simulink model "Sir_"  (R2015a)
settings: Solver=ode15s  StartTime=0.0  StopTime=10.0  RelTol=1e-3
libraries: fl_lib x20, elec_lib x9, nesl_utility x4, slctrlblks x1
settings Model: Creator=Ferdous  LastModifiedBy=joypc

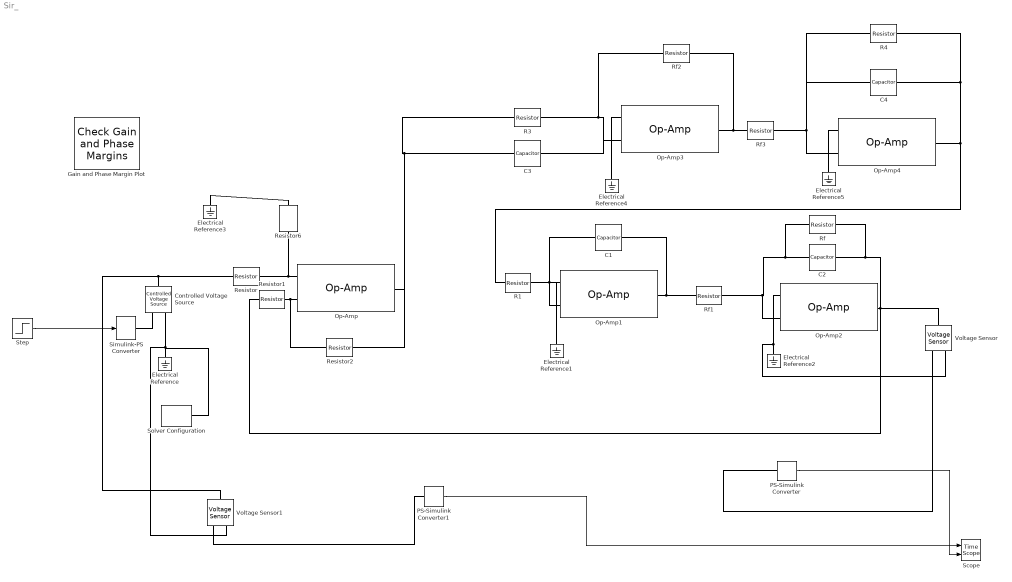
== system Sir_ ==
  C1 : fl_lib/Electrical/Electrical Elements/Capacitor  c=1e-6 F  r=1e-6 Ohm  g=0 1/Ohm  i_specify=off  i_priority=High  i=0 A  v_specify=off  v_priority=High  v=0 V  vc_specify=off  vc_priority=High  vc=0 V
  C2 : fl_lib/Electrical/Electrical Elements/Capacitor  c=0.122255367 F  r=1e-6 Ohm  g=0 1/Ohm  i_specify=off  i_priority=High  i=0 A  v_specify=off  v_priority=High  v=0 V  vc_specify=off  vc_priority=High  vc=0 V
  C3 : fl_lib/Electrical/Electrical Elements/Capacitor  c=2.51154 F  r=1e-6 Ohm  g=0 1/Ohm  i_specify=off  i_priority=High  i=0 A  v_specify=off  v_priority=High  v=0 V  vc_specify=off  vc_priority=High  vc=0 V
  C4 : fl_lib/Electrical/Electrical Elements/Capacitor  c=1.56 F  r=1e-6 Ohm  g=0 1/Ohm  i_specify=off  i_priority=High  i=0 A  v_specify=off  v_priority=High  v=0 V  vc_specify=off  vc_priority=High  vc=0 V
  Controlled Voltage Source : fl_lib/Electrical/Electrical Sources/Controlled Voltage Source
  Electrical Reference{,1..5} (6 alike) : fl_lib/Electrical/Electrical Elements/Electrical Reference
  Gain and Phase Margin Plot : slctrlblks/Model Verification/Check Gain and Phase Margins  InstantiateOnLoad=on  SaveOperatingPoints=off  LinearizationIOs={'/Step', 1, 'in', 'off', '';'/PS-Simulink Converter', 1, 'out', 'on', ''}  LinearizeAt=SnapshotTimes  SnapshotTimes=[0]  TriggerType=rising  SampleTime=auto  RateConversionMethod=zoh  PreWarpFreq=10  UseExactDelayModel=off  UseFullBlockNameLabels=off  UseBusSignalLabels=off  enabled=on  stopWhenAssertionFail=off  export=off  ViewDlgPos=[100 200 510 390]  LaunchViewOnOpen=off  OpenViewOnLoad=off  FrequencyUnits=rad/s  MagnitudeUnits=dB  PhaseUnits=deg  TimeUnits=seconds  EnableMargins=off  GainMargin=[]  PhaseMargin=[]  PlotType=bode  FeedbackSign=-1
      settings: SaveToWorkspace=off  SaveName=sys
  Op-Amp{,1..4} (5 alike) : fl_lib/Electrical/Electrical Elements/Op-Amp  outI_specify=off  outI_priority=High  outI=0 A
  PS-Simulink Converter : nesl_utility/PS-Simulink Converter  PhysicalDomain=network_engine_domain  SubClassName=ps_output  LeftPortType=input  RightPortType=output  PseudoPeriodic=off  Frequencies=[]  Unit=1  AffineConversion=off
  PS-Simulink Converter1 : nesl_utility/PS-Simulink Converter  PhysicalDomain=network_engine_domain  SubClassName=ps_output  LeftPortType=input  RightPortType=output  PseudoPeriodic=off  Frequencies=[]  Unit=1  AffineConversion=off
  R1 : elec_lib/Passive Devices/Resistor  R=1 kOhm  noise_mode=0  Tdevice=25 C  sample_time=0.001 s  repeatability=1  auto_seed=2279758131  user_seed=0
  R3 : elec_lib/Passive Devices/Resistor  R=0.995584 Ohm  noise_mode=0  Tdevice=25 C  sample_time=0.001 s  repeatability=1  auto_seed=1450493821  user_seed=0
  "R4 " : elec_lib/Passive Devices/Resistor  R=2.58816 Ohm  noise_mode=0  Tdevice=25 C  sample_time=0.001 s  repeatability=1  auto_seed=3865701835  user_seed=0
  Resistor : fl_lib/Electrical/Electrical Elements/Resistor  R=1 kOhm  i_specify=off  i_priority=High  i=0 A  v_specify=off  v_priority=High  v=0 V
  Resistor1 : fl_lib/Electrical/Electrical Elements/Resistor  R=1 kOhm  i_specify=off  i_priority=High  i=0 A  v_specify=off  v_priority=High  v=0 V
  Resistor2 : elec_lib/Passive Devices/Resistor  R=1 kOhm  noise_mode=0  Tdevice=25 C  sample_time=0.001 s  repeatability=1  auto_seed=1092133643  user_seed=0
  Resistor6 : elec_lib/Passive Devices/Resistor  R=1 kOhm  noise_mode=0  Tdevice=25 C  sample_time=0.001 s  repeatability=1  auto_seed=1585902849  user_seed=0
  Rf : elec_lib/Passive Devices/Resistor  R=5.107142857 Ohm  noise_mode=0  Tdevice=25 C  sample_time=0.001 s  repeatability=1  auto_seed=654458608  user_seed=0
  Rf1 : elec_lib/Passive Devices/Resistor  R=1 kOhm  noise_mode=0  Tdevice=25 C  sample_time=0.001 s  repeatability=1  auto_seed=3346497771  user_seed=0
  Rf2 : elec_lib/Passive Devices/Resistor  R=1 Ohm  noise_mode=0  Tdevice=25 C  sample_time=0.001 s  repeatability=1  auto_seed=1585902849  user_seed=0
  Rf3 : elec_lib/Passive Devices/Resistor  R=1 Ohm  noise_mode=0  Tdevice=25 C  sample_time=0.001 s  repeatability=1  auto_seed=477612198  user_seed=0
  Scope : TimeScope  NumInputPorts=2
  Simulink-PS Converter : nesl_utility/Simulink-PS Converter  PhysicalDomain=network_engine_domain  SubClassName=ps_input  LeftPortType=input  RightPortType=output  PseudoPeriodic=off  Frequencies=[]  NoiseDistribution=none  NoiseParameters=[]  Unit=1  AffineConversion=off  InputFiltering=off  SimscapeFilterOrder=1  InputFilterTimeConstant=0.001  UdotUserProvided=1
  Solver Configuration : nesl_utility/Solver Configuration  PhysicalDomain=network_engine_domain  SubClassName=solver  LeftPortType=input  RightPortType=generic  Accelerate=off  Tones=[]  Harmonics=[]  SimulateNoise=off  Profile=off  UseLocalSampling=off  EnableSwitchedLinearOptims=on  FrequencyDomain=off  UseCCode=off  RelTol=0.001  AbsTol=1e-06  MinStep=1e-09  ToWorkspace=off  RevertToSquareIcSolve=off  NumHomotopyIterations=100  DoDC=off  ResidualTolerance=1e-09  UseLocalSolver=off  LocalSolverChoice=NE_BACKWARD_EULER_ADVANCER  LocalSolverSampleTime=0.001  DoFixedCost=off  MaxNonlinIter=3  MaxModeIter=2  LinearAlgebra=Sparse  DelaysMemoryBudget=1024  AutomaticFiltering=on  FilteringTimeConstant=0.001
  Step : Step  SampleTime=0
  Voltage Sensor : fl_lib/Electrical/Electrical Sensors/Voltage Sensor
  Voltage Sensor1 : fl_lib/Electrical/Electrical Sensors/Voltage Sensor
  wires:
  Step/1 -> Simulink-PS Converter/1
  PS-Simulink Converter1/1 -> Scope/1
  PS-Simulink Converter/1 -> Scope/2
  connections:
  Resistor/RConn1 -- Resistor6/LConn1 -- Op-Amp/LConn1
  Resistor1/LConn1 -- Resistor2/LConn1 -- Op-Amp/LConn2
  Controlled Voltage Source/LConn1 -- Voltage Sensor1/LConn1 -- Resistor/LConn1
  Electrical Reference/LConn1 -- Controlled Voltage Source/RConn2 -- Solver Configuration/RConn1 -- Voltage Sensor1/RConn2
  Simulink-PS Converter/RConn1 -- Controlled Voltage Source/RConn1
  R1/RConn1 -- C1/LConn1 -- Op-Amp1/LConn2
  Rf1/LConn1 -- Op-Amp1/RConn1 -- C1/RConn1
  Rf1/RConn1 -- Op-Amp2/LConn2 -- Rf/LConn1 -- C2/LConn1
  C2/RConn1 -- Rf/RConn1 -- Voltage Sensor/LConn1 -- Op-Amp2/RConn1 -- Resistor1/RConn1
  Op-Amp1/LConn1 -- Electrical Reference1/LConn1
  Electrical Reference2/LConn1 -- Voltage Sensor/RConn2 -- Op-Amp2/LConn1
  Voltage Sensor1/RConn1 -- PS-Simulink Converter1/LConn1
  Voltage Sensor/RConn1 -- PS-Simulink Converter/LConn1
  Electrical Reference3/LConn1 -- Resistor6/RConn1
  Rf2/LConn1 -- R3/RConn1 -- Op-Amp3/LConn2 -- C3/RConn1
  Op-Amp3/RConn1 -- Rf2/RConn1 -- Rf3/LConn1
  Rf3/RConn1 -- Op-Amp4/LConn2 -- "R4 "/LConn1 -- C4/LConn1
  "R4 "/RConn1 -- C4/RConn1 -- R1/LConn1 -- Op-Amp4/RConn1
  C3/LConn1 -- Resistor2/RConn1 -- Op-Amp/RConn1 -- R3/LConn1
  Op-Amp4/LConn1 -- Electrical Reference5/LConn1
  Op-Amp3/LConn1 -- Electrical Reference4/LConn1
